simulink model "EKFsimu"  (R2021a)
settings: Solver=VariableStepAuto  StartTime=0.0  StopTime=10.0  RelTol=1e-3
values from neighbouring files (symbols this model uses):
  xkload = timeseries(xk(:,250:350),0:0.1:10)    [RunMe.m]
settings Model: Creator=Simão Amaro  LastModifiedBy=simao

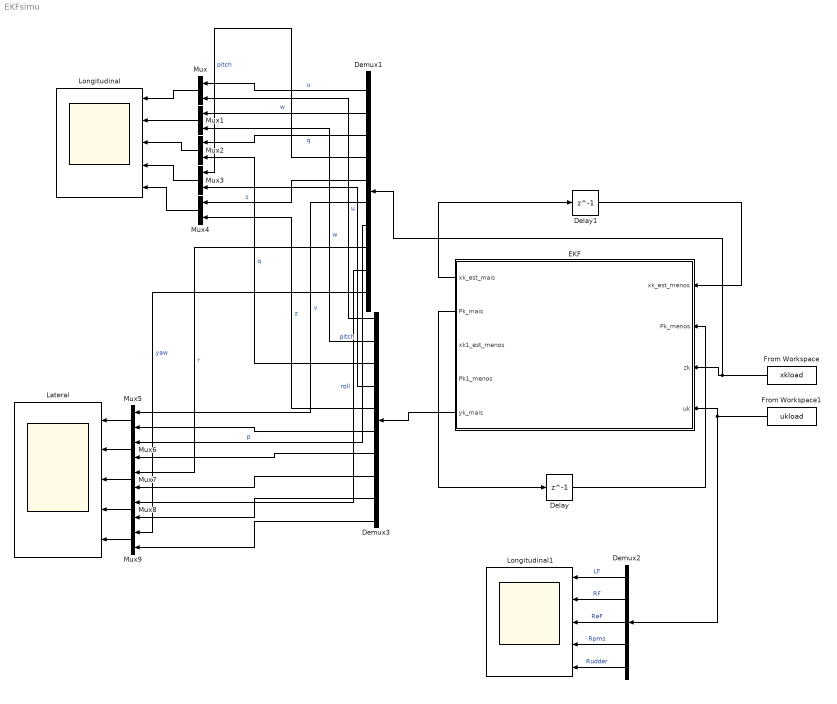
== system EKFsimu ==
  Delay : Delay  DelayLength=1  InitialCondition=10*eye(10)  SampleTime=0.02
  Delay1 : Delay  DelayLength=1  InitialCondition=xkload.Data(:,1,1)  SampleTime=0.02
  Demux1 : Demux  Outputs=10
  Demux2 : Demux  Outputs=5
  Demux3 : Demux  Outputs=10
  EKF : MATLAB Function  TreatAsAtomicUnit=on
  From Workspace : FromWorkspace  VariableName=xkload  SampleTime=0.1
  From Workspace1 : FromWorkspace  VariableName=ukload  SampleTime=0.1
  Lateral : Scope  NumInputPorts=5
  Longitudinal : Scope  NumInputPorts=5
  Longitudinal1 : Scope  NumInputPorts=5
  Mux{,1..9} (10 alike) : Mux  Inputs=2
  wires:
  EKF/1(xk_est_mais) -> Delay1/1
  Delay1/1 -> EKF/1(xk_est_menos)
  EKF/2(Pk_mais) -> Delay/1
  Delay/1 -> EKF/2(Pk_menos)
  From Workspace/1 -> Demux1/1, EKF/3(zk)
  From Workspace1/1 -> Demux2/1, EKF/4(uk)
  EKF/5(yk_mais) -> Demux3/1
  Mux/1 -> Longitudinal/1
  Mux1/1 -> Longitudinal/2
  Mux2/1 -> Longitudinal/3
  Mux3/1 -> Longitudinal/4
  Mux4/1 -> Longitudinal/5
  Demux1/1 -> Mux/1  "u"
  Demux3/1 -> Mux/2  "u"
  Demux3/2 -> Mux1/2  "w"
  Demux1/2 -> Mux1/1  "w"
  Demux3/3 -> Mux2/2  "q"
  Demux3/4 -> Mux3/2  "pitch"
  Demux3/5 -> Mux4/2  "z"
  Demux1/3 -> Mux2/1  "q"
  Demux1/4 -> Mux3/1  "pitch"
  Demux1/5 -> Mux4/1  "z"
  Mux5/1 -> Lateral/1
  Mux6/1 -> Lateral/2
  Mux7/1 -> Lateral/3
  Mux8/1 -> Lateral/4
  Mux9/1 -> Lateral/5
  Demux3/6 -> Mux5/2
  Demux3/7 -> Mux6/2
  Demux3/8 -> Mux7/2
  Demux3/10 -> Mux9/2
  Demux1/6 -> Mux5/1  "v"
  Demux1/7 -> Mux6/1  "p"
  Demux1/8 -> Mux7/1  "r"
  Demux1/9 -> Mux8/1  "roll"
  Demux1/10 -> Mux9/1  "yaw"
  Demux2/1 -> Longitudinal1/1  "LF"
  Demux2/2 -> Longitudinal1/2  "RF"
  Demux2/3 -> Longitudinal1/3  "ReF"
  Demux2/4 -> Longitudinal1/4  "Rpms"
  Demux2/5 -> Longitudinal1/5  "Rudder"
  Demux3/9 -> Mux8/2

== matlab function EKFsimu/EKF ==
  data: xk_est_mais output; xk_est_menos input; Pk_menos input; zk input; Pk_mais output; xk1_est_menos output; Pk1_menos output; uk input; yk_mais output
function [xk_est_mais,Pk_mais,xk1_est_menos,Pk1_menos,yk_mais] = extended_kalman_filter(xk_est_menos,Pk_menos,zk,uk)

%EKF matrices
Rk = diag([0.0005^2 0.0005^2 0.05^2 0.0005^2 0.00005^2 0.0005^2 0.05^2 0.05^2 0.005^2 0.005^2]); 
Qku = 0.0001*eye(10); %Quando tiver erro de modelo
%Qku = zeros(10,10);
%% RKM Aproximation

%Prediction Phase
%Phik = Jacobian_func_out(xk_est_menos(1),xk_est_menos(2),xk_est_menos(3),xk_est_menos(4),xk_est_menos(5),xk_est_menos(6),xk_est_menos(7),xk_est_menos(8),xk_est_menos(9),uk(3),uk(2),uk(1),uk(4),uk(5));
Phik = fwjac(xk_est_menos,uk);
Phik = expm(Phik*0.02);
Qk = Phik*Qku*Phik'*0.02;
xk1_est_menos = RKM_EKF(xk_est_menos,uk,0.02);
Pk1_menos = Phik*Pk_menos*Phik'+Qk;

%Correction Phase
yk = xk1_est_menos;
dist_cm_Us_x = 3.150;
Hk = Hk_func(xk1_est_menos(4),xk1_est_menos(5),xk1_est_menos(9));
yk(5) = (yk(5)*cosd(yk(9))-tand(yk(4))*dist_cm_Us_x)/cosd(yk(4)); 
Kk = Pk1_menos*Hk'*inv(Hk*Pk1_menos*Hk'+Rk);
xk_est_mais = xk1_est_menos+Kk*(zk-yk);
yk_mais = xk_est_mais;
yk_mais(5) = (yk_mais(5)*cosd(yk_mais(9))-tand(yk_mais(4))*dist_cm_Us_x)/cosd(yk_mais(4)); 
Pk_mais = (eye(10)-Kk*Hk)*Pk1_menos*(eye(10)-Kk*Hk)'+Kk*Rk*Kk';
end
